simulink model "lab5"  (R2019b)
settings: Solver=VariableStepAuto  StartTime=0.0  StopTime=100  RelTol=1e-3
settings Model: Creator=theojanson  LastModifiedBy=theojanson

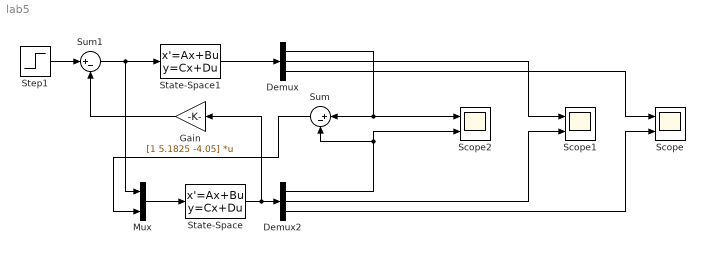
== system lab5 ==
  Demux : Demux  Outputs=3
  Demux2 : Demux  Outputs=3
  Gain : Gain  Gain=[1 5.1825 -4.05]  Multiplication=Matrix(K*u)
  Mux : Mux  Inputs=2
  Scope : Scope  NumInputPorts=2
  Scope1 : Scope  NumInputPorts=2
  Scope2 : Scope  NumInputPorts=2
  State-Space : StateSpace  A=[0 1 0 ; 0 -0.1 2 ; 0 -0.04 -20]  B=[0 0.0699e3 ; 0 1.3929e3; 0.002e3 5.998e3]  C=eye(3)  D=[0 0 ; 0 0 ; 0 0]  InitialCondition=0
  State-Space1 : StateSpace  A=[0 1 0 ; 0 -0.1 2 ; 0 -0.04 -20]  B=[0;0;2]  C=eye(3)  D="[0 ; 0  ; 0 ]"  InitialCondition=[3;4;5]
  Step1 : Step  SampleTime=0
  Sum : Sum  Inputs=|+-
  Sum1 : Sum  Inputs=|+-
  wires:
  Step1/1 -> Sum1/1
  Sum1/1 -> Mux/1, State-Space1/1
  State-Space1/1 -> Demux/1
  Gain/1 -> Sum1/2
  State-Space/1 -> Gain/1, Demux2/1
  Mux/1 -> State-Space/1
  Demux/1 -> Sum/1, Scope2/1
  Demux2/1 -> Sum/2, Scope2/2
  Sum/1 -> Mux/2
  Demux/2 -> Scope1/1
  Demux2/2 -> Scope1/2
  Demux2/3 -> Scope/2
  Demux/3 -> Scope/1
